simulink model "sampleModel7293_pp_1_1"  (R2018a)
settings: Solver=VariableStepAuto  StartTime=0.0  StopTime=10.0  RelTol=1e-3
undefined symbols (not defined in the file): DiscIntNeverNeededParam
libraries: simulink x367
(part 9 of 9)

== system sampleModel7293_pp_1_1/cfblk209/cfblk9 ==
  cfblk1 : Inport
  cfblk15 : Inport  Port=2
  Action Port : ActionPort  ActionType=then
  cfblk10 : simulink/Discrete/Difference  ICPrevInput=0.0  OutMin=[]  OutMax=[]  OutDataTypeStr=double  OutputDataTypeScalingMode=double  OutDataType=fixdt(1, 16)  OutScaling=2^-10  DoSatur=off
  cfblk11 : UnitDelay  SampleTime=-1
  cfblk12 : Delay
  cfblk13 : DiscreteStateSpace  SampleTime=-1
  cfblk14 : simulink/Discrete/Transfer Fcn Lead or Lag  PoleZ=0.95  ZeroZ=0.75  ICPrevOutput=0.0  ICPrevInput=0.0  DoSatur=off
      settings: SourceProductName=Simulink  SourceProductBaseCode=SL
  cfblk17 : Delay
  cfblk18 : Delay
  cfblk3 : simulink/Discrete/Transfer Fcn Lead or Lag  PoleZ=0.95  ZeroZ=0.75  ICPrevOutput=0.0  ICPrevInput=0.0  DoSatur=off
      settings: SourceProductName=Simulink  SourceProductBaseCode=SL
  cfblk4 : simulink/Discrete/Transfer Fcn First Order  PoleZ=0.95  ICPrevOutput=0.0  DoSatur=off
      settings: SourceProductName=Simulink
  cfblk5 : DiscreteIntegrator  SampleTime=-1  OutDataTypeStr=double  ICPrevOutput=DiscIntNeverNeededParam  ICPrevScaledInput=DiscIntNeverNeededParam
  cfblk6 : simulink/Discrete/Transfer Fcn Real Zero  ZeroZ=0.75  ICPrevInput=0.0  DoSatur=off
      settings: SourceProductName=Simulink  SourceProductBaseCode=SL
  cfblk7 : simulink/Discrete/Tapped Delay  vinit=0.0  samptime=-1  NumDelays=1  DelayOrder=Oldest  includeCurrent=off
  cfblk8 : simulink/Continuous/PID Controller  Controller=PID  TimeDomain=Discrete-time  SampleTime=-1  IntegratorMethod=Forward Euler  FilterMethod=Forward Euler  Form=Parallel  UseFilter=on  ControllerParametersSource=internal  P=1  I=1  D=0  N=100  InitialConditionSource=internal  InitialConditionForIntegrator=0  InitialConditionForFilter=0  ExternalReset=none  LimitOutput=off  UpperSaturationLimit=inf  LowerSaturationLimit=-inf  LinearizeAsGain=off  AntiWindupMode=none  Kb=1  TrackingMode=off  Kt=1  PParamMin=[]  PParamMax=[]  IParamMin=[]  IParamMax=[]  DParamMin=[]  DParamMax=[]  NParamMin=[]  NParamMax=[]  KbParamMin=[]  KbParamMax=[]  KtParamMin=[]  KtParamMax=[]  POutMin=[]  POutMax=[]  IOutMin=[]  IOutMax=[]  DOutMin=[]  DOutMax=[]  NOutMin=[]  NOutMax=[]  KbOutMin=[]  KbOutMax=[]  KtOutMin=[]  KtOutMax=[]  IntegratorOutMin=[]  IntegratorOutMax=[]  FilterOutMin=[]  FilterOutMax=[]  SumOutMin=[]  SumOutMax=[]  SumI1OutMin=[]  SumI1OutMax=[]  SumI2OutMin=[]  SumI2OutMax=[]  SumI3OutMin=[]  SumI3OutMax=[]  SumDOutMin=[]  SumDOutMax=[]  SaturationOutMin=[]  SaturationOutMax=[]  IntegratorContinuousStateAttributes=''  IntegratorStateMustResolveToSignalObject=off  IntegratorRTWStateStorageClass=Auto  FilterContinuousStateAttributes=''  FilterStateMustResolveToSignalObject=off  FilterRTWStateStorageClass=Auto  DifferentiatorICPrevScaledInput=0  DifferentiatorOutMin=[]  DifferentiatorOutMax=[]  FilterDiffOutCoefMin=[]  FilterDiffOutCoefMax=[]  SumDenOutMin=[]  SumDenOutMax=[]  SumNumOutMin=[]  SumNumOutMax=[]  ReciprocalOutMin=[]  ReciprocalOutMax=[]  DivideOutMin=[]  DivideOutMax=[]  TunerSelectOption=Transfer Function Based (PID Tuner App)
  cfblk9 : DiscreteFilter
  cyemi_{1353..1366} (14 alike) : DataTypeConversion  OutDataTypeStr=double
  cfblk2 : Outport
  cfblk16 : Outport  Port=2
  wires:
  cfblk1/1 -> cfblk16/1
  cfblk11/1 -> cfblk2/1
  cyemi_1353/1 -> cfblk10/1
  cfblk18/1 -> cyemi_1353/1
  cyemi_1354/1 -> cfblk11/1
  cfblk4/1 -> cyemi_1354/1
  cyemi_1355/1 -> cfblk12/1
  cfblk5/1 -> cyemi_1355/1
  cyemi_1356/1 -> cfblk13/1
  cfblk10/1 -> cyemi_1356/1
  cyemi_1357/1 -> cfblk14/1
  cfblk9/1 -> cyemi_1357/1
  cyemi_1358/1 -> cfblk17/1
  cfblk7/1 -> cyemi_1358/1
  cyemi_1359/1 -> cfblk18/1
  cfblk13/1 -> cyemi_1359/1
  cyemi_1360/1 -> cfblk3/1
  cfblk17/1 -> cyemi_1360/1
  cyemi_1361/1 -> cfblk4/1
  cfblk8/1 -> cyemi_1361/1
  cyemi_1362/1 -> cfblk5/1
  cfblk3/1 -> cyemi_1362/1
  cyemi_1363/1 -> cfblk6/1
  cfblk15/1 -> cyemi_1363/1
  cyemi_1364/1 -> cfblk7/1
  cfblk12/1 -> cyemi_1364/1
  cyemi_1365/1 -> cfblk8/1
  cfblk14/1 -> cyemi_1365/1
  cyemi_1366/1 -> cfblk9/1
  cfblk6/1 -> cyemi_1366/1

== system sampleModel7293_pp_1_1/cfblk210/cfblk17 ==
  cfblk1 : Inport
  cfblk8 : Inport  Port=2
  Action Port : ActionPort  ActionType=then
  cfblk3 : simulink/Discrete/Tapped Delay  vinit=0.0  samptime=-1  NumDelays=1  DelayOrder=Oldest  includeCurrent=off
  cfblk4 : Delay
  cfblk5 : Delay
  cfblk6 : simulink/Discrete/Tapped Delay  vinit=0.0  samptime=-1  NumDelays=1  DelayOrder=Oldest  includeCurrent=off
  cfblk7 : simulink/Discrete/Difference  ICPrevInput=0.0  OutMin=[]  OutMax=[]  OutDataTypeStr=double  OutputDataTypeScalingMode=double  OutDataType=fixdt(1, 16)  OutScaling=2^-10  DoSatur=off
  cyemi_{1378..1382} (5 alike) : DataTypeConversion  OutDataTypeStr=double
  cfblk2 : Outport
  wires:
  cfblk6/1 -> cfblk2/1
  cyemi_1378/1 -> cfblk3/1
  cfblk1/1 -> cyemi_1378/1
  cyemi_1379/1 -> cfblk4/1
  cfblk7/1 -> cyemi_1379/1
  cyemi_1380/1 -> cfblk5/1
  cfblk3/1 -> cyemi_1380/1
  cyemi_1381/1 -> cfblk6/1
  cfblk4/1 -> cyemi_1381/1
  cyemi_1382/1 -> cfblk7/1
  cfblk8/1 -> cyemi_1382/1

== system sampleModel7293_pp_1_1/cfblk210/cfblk18 ==
  cfblk1 : Inport
  cfblk12 : Inport  Port=2
  cfblk13 : Inport  Port=3
  Action Port : ActionPort  ActionType=else
  cfblk10 : simulink/Discrete/Transfer Fcn First Order  PoleZ=0.95  ICPrevOutput=0.0  DoSatur=off
      settings: SourceProductName=Simulink
  cfblk11 : UnitDelay  SampleTime=-1
  cfblk3 : simulink/Discrete/Transfer Fcn Real Zero  ZeroZ=0.75  ICPrevInput=0.0  DoSatur=off
      settings: SourceProductName=Simulink  SourceProductBaseCode=SL
  cfblk4 : simulink/Continuous/PID Controller  Controller=PID  TimeDomain=Discrete-time  SampleTime=-1  IntegratorMethod=Forward Euler  FilterMethod=Forward Euler  Form=Parallel  UseFilter=on  ControllerParametersSource=internal  P=1  I=1  D=0  N=100  InitialConditionSource=internal  InitialConditionForIntegrator=0  InitialConditionForFilter=0  ExternalReset=none  LimitOutput=off  UpperSaturationLimit=inf  LowerSaturationLimit=-inf  LinearizeAsGain=off  AntiWindupMode=none  Kb=1  TrackingMode=off  Kt=1  PParamMin=[]  PParamMax=[]  IParamMin=[]  IParamMax=[]  DParamMin=[]  DParamMax=[]  NParamMin=[]  NParamMax=[]  KbParamMin=[]  KbParamMax=[]  KtParamMin=[]  KtParamMax=[]  POutMin=[]  POutMax=[]  IOutMin=[]  IOutMax=[]  DOutMin=[]  DOutMax=[]  NOutMin=[]  NOutMax=[]  KbOutMin=[]  KbOutMax=[]  KtOutMin=[]  KtOutMax=[]  IntegratorOutMin=[]  IntegratorOutMax=[]  FilterOutMin=[]  FilterOutMax=[]  SumOutMin=[]  SumOutMax=[]  SumI1OutMin=[]  SumI1OutMax=[]  SumI2OutMin=[]  SumI2OutMax=[]  SumI3OutMin=[]  SumI3OutMax=[]  SumDOutMin=[]  SumDOutMax=[]  SaturationOutMin=[]  SaturationOutMax=[]  IntegratorContinuousStateAttributes=''  IntegratorStateMustResolveToSignalObject=off  IntegratorRTWStateStorageClass=Auto  FilterContinuousStateAttributes=''  FilterStateMustResolveToSignalObject=off  FilterRTWStateStorageClass=Auto  DifferentiatorICPrevScaledInput=0  DifferentiatorOutMin=[]  DifferentiatorOutMax=[]  FilterDiffOutCoefMin=[]  FilterDiffOutCoefMax=[]  SumDenOutMin=[]  SumDenOutMax=[]  SumNumOutMin=[]  SumNumOutMax=[]  ReciprocalOutMin=[]  ReciprocalOutMax=[]  DivideOutMin=[]  DivideOutMax=[]  TunerSelectOption=Transfer Function Based (PID Tuner App)
  cfblk5 : DiscreteIntegrator  SampleTime=-1  OutDataTypeStr=double  ICPrevOutput=DiscIntNeverNeededParam  ICPrevScaledInput=DiscIntNeverNeededParam
  cfblk6 : DiscreteZeroPole  Poles=[0 0.5]  Gain=1  SampleTime=-1
  cfblk7 : DiscreteFir
  cfblk8 : UnitDelay  SampleTime=-1
  cfblk9 : simulink/Discrete/Transfer Fcn Lead or Lag  PoleZ=0.95  ZeroZ=0.75  ICPrevOutput=0.0  ICPrevInput=0.0  DoSatur=off
      settings: SourceProductName=Simulink  SourceProductBaseCode=SL
  cyemi_{1386..1394} (9 alike) : DataTypeConversion  OutDataTypeStr=double
  cfblk2 : Outport
  wires:
  cfblk3/1 -> cfblk2/1
  cyemi_1386/1 -> cfblk10/1
  cfblk5/1 -> cyemi_1386/1
  cyemi_1387/1 -> cfblk11/1
  cfblk8/1 -> cyemi_1387/1
  cyemi_1388/1 -> cfblk3/1
  cfblk13/1 -> cyemi_1388/1
  cyemi_1389/1 -> cfblk4/1
  cfblk9/1 -> cyemi_1389/1
  cyemi_1390/1 -> cfblk5/1
  cfblk11/1 -> cyemi_1390/1
  cyemi_1391/1 -> cfblk6/1
  cfblk12/1 -> cyemi_1391/1
  cyemi_1392/1 -> cfblk7/1
  cfblk1/1 -> cyemi_1392/1
  cyemi_1393/1 -> cfblk8/1
  cfblk4/1 -> cyemi_1393/1
  cyemi_1394/1 -> cfblk9/1
  cfblk6/1 -> cyemi_1394/1

== system sampleModel7293_pp_1_1/cfblk213/cfblk14 ==
  cfblk1 : Inport
  cfblk13 : Inport  Port=2
  cfblk14 : Inport  Port=3
  Action Port : ActionPort  ActionType=then
  cfblk10 : simulink/Continuous/PID Controller  Controller=PID  TimeDomain=Discrete-time  SampleTime=-1  IntegratorMethod=Forward Euler  FilterMethod=Forward Euler  Form=Parallel  UseFilter=on  ControllerParametersSource=internal  P=1  I=1  D=0  N=100  InitialConditionSource=internal  InitialConditionForIntegrator=0  InitialConditionForFilter=0  ExternalReset=none  LimitOutput=off  UpperSaturationLimit=inf  LowerSaturationLimit=-inf  LinearizeAsGain=off  AntiWindupMode=none  Kb=1  TrackingMode=off  Kt=1  PParamMin=[]  PParamMax=[]  IParamMin=[]  IParamMax=[]  DParamMin=[]  DParamMax=[]  NParamMin=[]  NParamMax=[]  KbParamMin=[]  KbParamMax=[]  KtParamMin=[]  KtParamMax=[]  POutMin=[]  POutMax=[]  IOutMin=[]  IOutMax=[]  DOutMin=[]  DOutMax=[]  NOutMin=[]  NOutMax=[]  KbOutMin=[]  KbOutMax=[]  KtOutMin=[]  KtOutMax=[]  IntegratorOutMin=[]  IntegratorOutMax=[]  FilterOutMin=[]  FilterOutMax=[]  SumOutMin=[]  SumOutMax=[]  SumI1OutMin=[]  SumI1OutMax=[]  SumI2OutMin=[]  SumI2OutMax=[]  SumI3OutMin=[]  SumI3OutMax=[]  SumDOutMin=[]  SumDOutMax=[]  SaturationOutMin=[]  SaturationOutMax=[]  IntegratorContinuousStateAttributes=''  IntegratorStateMustResolveToSignalObject=off  IntegratorRTWStateStorageClass=Auto  FilterContinuousStateAttributes=''  FilterStateMustResolveToSignalObject=off  FilterRTWStateStorageClass=Auto  DifferentiatorICPrevScaledInput=0  DifferentiatorOutMin=[]  DifferentiatorOutMax=[]  FilterDiffOutCoefMin=[]  FilterDiffOutCoefMax=[]  SumDenOutMin=[]  SumDenOutMax=[]  SumNumOutMin=[]  SumNumOutMax=[]  ReciprocalOutMin=[]  ReciprocalOutMax=[]  DivideOutMin=[]  DivideOutMax=[]  TunerSelectOption=Transfer Function Based (PID Tuner App)
  cfblk11 : DiscreteZeroPole  Poles=[0 0.5]  Gain=1  SampleTime=-1
  cfblk12 : Delay  DelayLengthSource=Input port
      settings: InputPortMap=u0,p1
  cfblk16 : Delay
  cfblk17 : Delay
  cfblk18 : DataTypeConversion  OutDataTypeStr=uint32
  cfblk19 : DataTypeConversion  OutDataTypeStr=double
  cfblk3 : Delay  DelayLengthSource=Input port
      settings: InputPortMap=u0,p1
  cfblk4 : simulink/Discrete/Tapped Delay  vinit=0.0  samptime=-1  NumDelays=1  DelayOrder=Oldest  includeCurrent=off
  cfblk5 : DiscreteFir
  cfblk6 : Delay  ShowEnablePort=on
      settings: InputPortMap=u0,e6
  cfblk7 : DiscreteIntegrator  SampleTime=-1  OutDataTypeStr=double  ICPrevOutput=DiscIntNeverNeededParam  ICPrevScaledInput=DiscIntNeverNeededParam
  cfblk8 : Delay
  cfblk9 : Delay  DelayLengthSource=Input port
      settings: InputPortMap=u0,p1
  cyemi_{1429..1445} (17 alike) : DataTypeConversion  OutDataTypeStr=double
  cyemi_1446 : DataTypeConversion  OutDataTypeStr=uint32
  cfblk2 : Outport
  cfblk15 : Outport  Port=2
  wires:
  cfblk3/1 -> cfblk15/1
  cfblk8/1 -> cfblk2/1
  cfblk1/1 -> cyemi_1442/1, cyemi_1444/1
  cfblk4/1 -> cyemi_1431/1, cyemi_1445/1
  cfblk9/1 -> cyemi_1432/1, cyemi_1437/1
  cyemi_1429/1 -> cfblk10/1
  cfblk17/1 -> cyemi_1429/1
  cyemi_1430/1 -> cfblk11/1
  cfblk10/1 -> cyemi_1430/1
  cyemi_1431/1 -> cfblk12/1
  cyemi_1432/1 -> cfblk12/2
  cyemi_1433/1 -> cfblk16/1
  cfblk12/1 -> cyemi_1433/1
  cyemi_1434/1 -> cfblk17/1
  cfblk11/1 -> cyemi_1434/1
  cyemi_1435/1 -> cfblk18/1
  cfblk5/1 -> cyemi_1435/1
  cyemi_1436/1 -> cfblk19/1
  cfblk7/1 -> cyemi_1436/1
  cyemi_1437/1 -> cfblk3/1
  cyemi_1438/1 -> cfblk3/2
  cfblk13/1 -> cyemi_1438/1
  cyemi_1439/1 -> cfblk4/1
  cfblk6/1 -> cyemi_1439/1
  cyemi_1440/1 -> cfblk5/1
  cfblk19/1 -> cyemi_1440/1
  cyemi_1441/1 -> cfblk6/1
  cfblk16/1 -> cyemi_1441/1
  cyemi_1442/1 -> cfblk6/2
  cyemi_1443/1 -> cfblk7/1
  cfblk14/1 -> cyemi_1443/1
  cyemi_1444/1 -> cfblk8/1
  cyemi_1445/1 -> cfblk9/1
  cyemi_1446/1 -> cfblk9/2
  cfblk18/1 -> cyemi_1446/1

== system sampleModel7293_pp_1_1/cfblk213/cfblk15 ==
  cfblk1 : Inport
  cfblk9 : Inport  Port=2
  Action Port : ActionPort  ActionType=else
  cfblk11 : Delay
  cfblk12 : Delay
  cfblk3 : DiscreteIntegrator  SampleTime=-1  OutDataTypeStr=double  ICPrevOutput=DiscIntNeverNeededParam  ICPrevScaledInput=DiscIntNeverNeededParam
  cfblk4 : UnitDelay  SampleTime=-1
  cfblk5 : Delay
  cfblk6 : UnitDelay  SampleTime=-1
  cfblk7 : simulink/Discrete/Tapped Delay  vinit=0.0  samptime=-1  NumDelays=1  DelayOrder=Oldest  includeCurrent=off
  cfblk8 : DiscreteZeroPole  Poles=[0 0.5]  Gain=1  SampleTime=-1
  cyemi_{1449..1456} (8 alike) : DataTypeConversion  OutDataTypeStr=double
  cfblk2 : Outport
  cfblk10 : Outport  Port=2
  wires:
  cfblk1/1 -> cfblk10/1
  cfblk8/1 -> cfblk2/1
  cyemi_1449/1 -> cfblk11/1
  cfblk6/1 -> cyemi_1449/1
  cyemi_1450/1 -> cfblk12/1
  cfblk5/1 -> cyemi_1450/1
  cyemi_1451/1 -> cfblk3/1
  cfblk11/1 -> cyemi_1451/1
  cyemi_1452/1 -> cfblk4/1
  cfblk12/1 -> cyemi_1452/1
  cyemi_1453/1 -> cfblk5/1
  cfblk4/1 -> cyemi_1453/1
  cyemi_1454/1 -> cfblk6/1
  cfblk3/1 -> cyemi_1454/1
  cyemi_1455/1 -> cfblk7/1
  cfblk9/1 -> cyemi_1455/1
  cyemi_1456/1 -> cfblk8/1
  cfblk7/1 -> cyemi_1456/1
